simulink model "RM3_Hydraulic_PTO"  (R2019b)
settings: Solver=ode14x  StartTime=0  StopTime=100  FixedStep=0.0025  MaxStep=0.0025  RelTol=1e-3  EnableMultiTasking=on
undefined symbols (not defined in the file or in its folder): body, DiscIntNeverNeededParam, pto
libraries: fl_lib x208, sh_lib x67, nesl_utility x67, WECSim_Lib x5
(part 5 of 5)

== system RM3_Hydraulic_PTO/PTO-Sim - Crankshaft DA 4 Cylinders Try 4 WORKS /Cylinder 3/Hydraulic cylinder and valves ==
  3 Way Directional Valve : sh_lib/Valves/Directional Valves/3-Way Directional Valve  area_spec=sh.valves.directional_valves.enum.area_spec.identical  x_0_P=0 m  x_0_T=0 m  mdl_type_identical=sh.valves.directional_valves.enum.mdl_type.linear  mdl_type_different=sh.valves.directional_valves.enum.mdl_type.linear  opening_max=0.75 in  area_max=pi*(0.75/2)^2 in^2  opening_max_P_A=0.005 m  area_max_P_A=0.5e-4 m^2  opening_max_A_T=0.005 m  area_max_A_T=0.5e-4 m^2  opening_area_tab=[-.002, 0, .002, .005, .015] m  area_tab=[1e-09, 2.0352e-07, 4.0736e-05, .00011438, .00034356] m^2  opening_flow_rate_tab=[-.002, 0, .002, .005, .015] m  pressure_tab=[-10000000, -5000000, -2000000, 2000000, 5000000, 10000000] Pa  flow_rate_tab=[-1e-07, -7.0711e-08, -4.4721e-08, 4.4721e-08, 7.0711e-08, 1e-07; -2.0352e-05, -1.4391e-05, -9.1017e-06, 9.1017e-06, 1.4391e-05, 2.0352e-05; -.0040736, -.0028805, -.0018218, .0018218, .0028805, .0040736; -.011438, -.0080879, -.0051152, .0051152, .0080879, .011438; -.034356, -.024293, -.015364, .015364, .024293, .034356] m^3/s  opening_area_tab_P_A=[-.002, 0, .002, .005, .015] m  area_tab_P_A=[1e-09, 2.0352e-07, 4.0736e-05, .00011438, .00034356] m^2  opening_flow_rate_tab_P_A=[-.002, 0, .002, .005, .015] m  pressure_tab_P_A=[-10000000, -5000000, -2000000, 2000000, 5000000, 10000000] Pa  flow_rate_tab_P_A=[-1e-07, -7.0711e-08, -4.4721e-08, 4.4721e-08, 7.0711e-08, 1e-07; -2.0352e-05, -1.4391e-05, -9.1017e-06, 9.1017e-06, 1.4391e-05, 2.0352e-05; -.0040736, -.0028805, -.0018218, .0018218, .0028805, .0040736; -.011438, -.0080879, -.0051152, .0051152, .0080879, .011438; -.034356, -.024293, -.015364, .015364, .024293, .034356] m^3/s  opening_area_tab_A_T=[-.002, 0, .002, .005, .015] m  area_tab_A_T=[1e-09, 2.0352e-07, 4.0736e-05, .00011438, .00034356] m^2  opening_flow_rate_tab_A_T=[-.002, 0, .002, .005, .015] m  pressure_tab_A_T=[-10000000, -5000000, -2000000, 2000000, 5000000, 10000000] Pa  flow_rate_tab_A_T=[-1e-07, -7.0711e-08, -4.4721e-08, 4.4721e-08, 7.0711e-08, 1e-07; -2.0352e-05, -1.4391e-05, -9.1017e-06, 9.1017e-06, 1.4391e-05, 2.0352e-05; -.0040736, -.0028805, -.0018218, .0018218, .0028805, .0040736; -.011438, -.0080879, -.0051152, .0051152, .0080879, .011438; -.034356, -.024293, -.015364, .015364, .024293, .034356] m^3/s  interp_method_identical=sh.valves.directional_valves.enum.interp_method.linear  interp_method_different=sh.valves.directional_valves.enum.interp_method.linear  extrap_method_identical=sh.valves.directional_valves.enum.extrap_method.linear  extrap_method_different=sh.valves.directional_valves.enum.extrap_method.linear  A_leak=1e-12 m^2  C_d=0.7  lam_spec=sh.valves.directional_valves.enum.lam_spec.pressure_ratio  B_lam=0.999  Re_cr=12
      settings: SourceProductName=Simscape Fluids  SourceProductBaseCode=SH  InternalSimscapePortConfiguration="{\"Bottom\":[],\"Left\":[{\"id\":\"A\",\"label\":\"A\",\"type\":\"foundation.hydraulic.hydraulic\"}],\"Right\":[{\"id\":\"S\",\"label\":\"S\",\"type\":\"input\"},{\"id\":\"P\",\"label\":\"P\",\"type\":\"foundation.hydraulic.hydraulic\"},{\"id\":\"T\",\"label\":\"T\",\"type\":\"foundation.hydraulic.hydraulic\"}],\"Top\":[]}"
  3 Way Directional Valve1 : sh_lib/Valves/Directional Valves/3-Way Directional Valve  area_spec=sh.valves.directional_valves.enum.area_spec.identical  x_0_P=0 m  x_0_T=0 m  mdl_type_identical=sh.valves.directional_valves.enum.mdl_type.linear  mdl_type_different=sh.valves.directional_valves.enum.mdl_type.linear  opening_max=0.75 in  area_max=pi*(0.75/2)^2 in^2  opening_max_P_A=0.005 m  area_max_P_A=0.5e-4 m^2  opening_max_A_T=0.005 m  area_max_A_T=0.5e-4 m^2  opening_area_tab=[-.002, 0, .002, .005, .015] m  area_tab=[1e-09, 2.0352e-07, 4.0736e-05, .00011438, .00034356] m^2  opening_flow_rate_tab=[-.002, 0, .002, .005, .015] m  pressure_tab=[-10000000, -5000000, -2000000, 2000000, 5000000, 10000000] Pa  flow_rate_tab=[-1e-07, -7.0711e-08, -4.4721e-08, 4.4721e-08, 7.0711e-08, 1e-07; -2.0352e-05, -1.4391e-05, -9.1017e-06, 9.1017e-06, 1.4391e-05, 2.0352e-05; -.0040736, -.0028805, -.0018218, .0018218, .0028805, .0040736; -.011438, -.0080879, -.0051152, .0051152, .0080879, .011438; -.034356, -.024293, -.015364, .015364, .024293, .034356] m^3/s  opening_area_tab_P_A=[-.002, 0, .002, .005, .015] m  area_tab_P_A=[1e-09, 2.0352e-07, 4.0736e-05, .00011438, .00034356] m^2  opening_flow_rate_tab_P_A=[-.002, 0, .002, .005, .015] m  pressure_tab_P_A=[-10000000, -5000000, -2000000, 2000000, 5000000, 10000000] Pa  flow_rate_tab_P_A=[-1e-07, -7.0711e-08, -4.4721e-08, 4.4721e-08, 7.0711e-08, 1e-07; -2.0352e-05, -1.4391e-05, -9.1017e-06, 9.1017e-06, 1.4391e-05, 2.0352e-05; -.0040736, -.0028805, -.0018218, .0018218, .0028805, .0040736; -.011438, -.0080879, -.0051152, .0051152, .0080879, .011438; -.034356, -.024293, -.015364, .015364, .024293, .034356] m^3/s  opening_area_tab_A_T=[-.002, 0, .002, .005, .015] m  area_tab_A_T=[1e-09, 2.0352e-07, 4.0736e-05, .00011438, .00034356] m^2  opening_flow_rate_tab_A_T=[-.002, 0, .002, .005, .015] m  pressure_tab_A_T=[-10000000, -5000000, -2000000, 2000000, 5000000, 10000000] Pa  flow_rate_tab_A_T=[-1e-07, -7.0711e-08, -4.4721e-08, 4.4721e-08, 7.0711e-08, 1e-07; -2.0352e-05, -1.4391e-05, -9.1017e-06, 9.1017e-06, 1.4391e-05, 2.0352e-05; -.0040736, -.0028805, -.0018218, .0018218, .0028805, .0040736; -.011438, -.0080879, -.0051152, .0051152, .0080879, .011438; -.034356, -.024293, -.015364, .015364, .024293, .034356] m^3/s  interp_method_identical=sh.valves.directional_valves.enum.interp_method.linear  interp_method_different=sh.valves.directional_valves.enum.interp_method.linear  extrap_method_identical=sh.valves.directional_valves.enum.extrap_method.linear  extrap_method_different=sh.valves.directional_valves.enum.extrap_method.linear  A_leak=1e-12 m^2  C_d=0.7  lam_spec=sh.valves.directional_valves.enum.lam_spec.pressure_ratio  B_lam=0.999  Re_cr=12
      settings: SourceProductName=Simscape Fluids  SourceProductBaseCode=SH  InternalSimscapePortConfiguration="{\"Bottom\":[],\"Left\":[{\"id\":\"A\",\"label\":\"A\",\"type\":\"foundation.hydraulic.hydraulic\"}],\"Right\":[{\"id\":\"S\",\"label\":\"S\",\"type\":\"input\"},{\"id\":\"P\",\"label\":\"P\",\"type\":\"foundation.hydraulic.hydraulic\"},{\"id\":\"T\",\"label\":\"T\",\"type\":\"foundation.hydraulic.hydraulic\"}],\"Top\":[]}"
  Check Valve : sh_lib/Valves/Directional Valves/Check Valve  Commented=on  area_max=pi*(0.75/2)^2 in^2  pres_crack=0.3e5 Pa  pres_max=1.2e5 Pa  C_d=0.7  A_leak=1e-12 m^2  lam_spec=1  B_lam=0.999  Re_cr=12  dynamic=0  tau=0.1 s  area_init=1e-12 m^2
      settings: SourceProductName=Simscape Fluids  SourceProductBaseCode=SH  InternalSimscapePortConfiguration="{\"Bottom\":[],\"Left\":[{\"id\":\"A\",\"label\":\"A\",\"type\":\"foundation.hydraulic.hydraulic\"}],\"Right\":[{\"id\":\"B\",\"label\":\"B\",\"type\":\"foundation.hydraulic.hydraulic\"}],\"Top\":[]}"
  Check Valve1 : sh_lib/Valves/Directional Valves/Check Valve  Commented=on  area_max=pi*(0.75/2)^2 in^2  pres_crack=0.3e5 Pa  pres_max=1.2e5 Pa  C_d=0.7  A_leak=1e-12 m^2  lam_spec=1  B_lam=0.999  Re_cr=12  dynamic=0  tau=0.1 s  area_init=1e-12 m^2
      settings: SourceProductName=Simscape Fluids  SourceProductBaseCode=SH  InternalSimscapePortConfiguration="{\"Bottom\":[],\"Left\":[{\"id\":\"A\",\"label\":\"A\",\"type\":\"foundation.hydraulic.hydraulic\"}],\"Right\":[{\"id\":\"B\",\"label\":\"B\",\"type\":\"foundation.hydraulic.hydraulic\"}],\"Top\":[]}"
  Double-Acting Hydraulic Cylinder (Simple) : sh_lib/Hydraulic Cylinders/Double-Acting Hydraulic Cylinder (Simple)  area_A=0.0025746658/4 m^2  area_B=0.0025746658/4 m^2  stroke=12 in  init_pos=5 in  penetr_coeff=1e12 s*N/m^2  or=1
      settings: SourceProductName=Simscape Fluids  SourceProductBaseCode=SH  InternalSimscapePortConfiguration="{\"Bottom\":[],\"Left\":[{\"id\":\"C\",\"label\":\"C\",\"type\":\"foundation.mechanical.translational.translational\"},{\"id\":\"A\",\"label\":\"A\",\"type\":\"foundation.hydraulic.hydraulic\"}],\"Right\":[{\"id\":\"R\",\"label\":\"R\",\"type\":\"foundation.mechanical.translational.translational\"},{\"id\":\"B\",\"label\":\"B\",\"type\":\"foundation.hydraulic.hydraulic\"}],\"Top\":[]}"
  Ideal Force Sensor : fl_lib/Mechanical/Mechanical Sensors/Ideal Force Sensor
  Ideal Translational Velocity Source : fl_lib/Mechanical/Mechanical Sources/Ideal Translational Velocity Source
  Mechanical Translational Reference : fl_lib/Mechanical/Translational Elements/Mechanical Translational Reference
  Mechanical Translational Reference1 : fl_lib/Mechanical/Translational Elements/Mechanical Translational Reference
  PS Gain : fl_lib/Physical Signals/Functions/PS Gain  gain=-1
  PS-Simulink Converter : nesl_utility/PS-Simulink Converter  PhysicalDomain=network_engine_domain  SubClassName=ps_output  LeftPortType=input  RightPortType=output  PseudoPeriodic=off  Frequencies=[]  Unit=N  AffineConversion=off
  PS-Simulink Converter2 : nesl_utility/PS-Simulink Converter  PhysicalDomain=network_engine_domain  SubClassName=ps_output  LeftPortType=input  RightPortType=output  PseudoPeriodic=off  Frequencies=[]  Unit=inherit  AffineConversion=off
  Relay : Relay  OnSwitchValue=0  OffSwitchValue=0  OffOutputValue=-1
  Simulink-PS Converter1 : nesl_utility/Simulink-PS Converter  PhysicalDomain=network_engine_domain  SubClassName=ps_input  LeftPortType=input  RightPortType=output  PseudoPeriodic=off  Frequencies=[]  NoiseDistribution=none  NoiseParameters=[]  Unit=1  AffineConversion=off  FilteringAndDerivatives=zero  SimscapeFilterOrder=1  InputFilterTimeConstant=0.001  UdotUserProvided=0
  Velocity input : PMIOPort  Side=Left
  Flow out : PMIOPort  Port=2  Side=Left
  Seawater In : PMIOPort  Port=3  Side=Left
  Force Out : Outport
  wires:
  PS-Simulink Converter2/1 -> Relay/1
  Relay/1 -> Simulink-PS Converter1/1
  PS-Simulink Converter/1 -> Force Out/1
  connections:
  Ideal Translational Velocity Source/LConn1 -- Double-Acting Hydraulic Cylinder (Simple)/RConn1
  3 Way Directional Valve1/RConn2 -- 3 Way Directional Valve/RConn2 -- Seawater In/RConn1
  3 Way Directional Valve/RConn3 -- 3 Way Directional Valve1/RConn3 -- Flow out/RConn1
  3 Way Directional Valve/LConn1 -- Double-Acting Hydraulic Cylinder (Simple)/LConn2
  Simulink-PS Converter1/RConn1 -- PS Gain/LConn1 -- 3 Way Directional Valve/RConn1
  Ideal Translational Velocity Source/RConn1 -- PS-Simulink Converter2/LConn1 -- Velocity input/RConn1
  Ideal Translational Velocity Source/RConn2 -- Mechanical Translational Reference1/LConn1
  Double-Acting Hydraulic Cylinder (Simple)/RConn2 -- 3 Way Directional Valve1/LConn1
  PS Gain/RConn1 -- 3 Way Directional Valve1/RConn1
  Ideal Force Sensor/RConn2 -- PS-Simulink Converter/LConn1
  Ideal Force Sensor/RConn1 -- Mechanical Translational Reference/LConn1
  Ideal Force Sensor/LConn1 -- Double-Acting Hydraulic Cylinder (Simple)/LConn1

== system RM3_Hydraulic_PTO/PTO-Sim - Crankshaft DA 4 Cylinders Try 4 WORKS /Cylinder 4/Cylinder 1 to PTO Force convert ==
  Crank radius : Inport
  Crank initial angle : Inport  Port=2
  Angle disp : Inport  Port=3
  Spool radius : Inport  Port=4
  Cylinder Force : Inport  Port=5
  Constant : Constant
  Divide1 : Product  Inputs=*/
  Mod angle : Constant  Value=2*pi
  PTO Force Cylinder 1 : Product  Inputs=4
  Sin(theta) : Trigonometry
  Sum : Sum  Inputs=|++
  To get Theta : Math  Operator=mod  SignedPower=off  SaturateOnIntegerOverflow=on
  Theta : Outport
  sing(theta) : Outport  Port=2
  PTO Force Cyl : Outport  Port=3
  wires:
  Mod angle/1 -> To get Theta/2
  Angle disp/1 -> Sum/2
  To get Theta/1 -> Theta/1, Sin(theta)/1
  PTO Force Cylinder 1/1 -> PTO Force Cyl/1
  Divide1/1 -> PTO Force Cylinder 1/3
  Sin(theta)/1 -> sing(theta)/1, PTO Force Cylinder 1/2
  Constant/1 -> Divide1/1
  Crank initial angle/1 -> Sum/1
  Sum/1 -> To get Theta/1
  Spool radius/1 -> Divide1/2
  Cylinder Force/1 -> PTO Force Cylinder 1/4
  Crank radius/1 -> PTO Force Cylinder 1/1

== system RM3_Hydraulic_PTO/PTO-Sim - Crankshaft DA 4 Cylinders Try 4 WORKS /Cylinder 4/Hydraulic cylinder and valves ==
  3 Way Directional Valve : sh_lib/Valves/Directional Valves/3-Way Directional Valve  area_spec=sh.valves.directional_valves.enum.area_spec.identical  x_0_P=0 m  x_0_T=0 m  mdl_type_identical=sh.valves.directional_valves.enum.mdl_type.linear  mdl_type_different=sh.valves.directional_valves.enum.mdl_type.linear  opening_max=0.75 in  area_max=pi*(0.75/2)^2 in^2  opening_max_P_A=0.005 m  area_max_P_A=0.5e-4 m^2  opening_max_A_T=0.005 m  area_max_A_T=0.5e-4 m^2  opening_area_tab=[-.002, 0, .002, .005, .015] m  area_tab=[1e-09, 2.0352e-07, 4.0736e-05, .00011438, .00034356] m^2  opening_flow_rate_tab=[-.002, 0, .002, .005, .015] m  pressure_tab=[-10000000, -5000000, -2000000, 2000000, 5000000, 10000000] Pa  flow_rate_tab=[-1e-07, -7.0711e-08, -4.4721e-08, 4.4721e-08, 7.0711e-08, 1e-07; -2.0352e-05, -1.4391e-05, -9.1017e-06, 9.1017e-06, 1.4391e-05, 2.0352e-05; -.0040736, -.0028805, -.0018218, .0018218, .0028805, .0040736; -.011438, -.0080879, -.0051152, .0051152, .0080879, .011438; -.034356, -.024293, -.015364, .015364, .024293, .034356] m^3/s  opening_area_tab_P_A=[-.002, 0, .002, .005, .015] m  area_tab_P_A=[1e-09, 2.0352e-07, 4.0736e-05, .00011438, .00034356] m^2  opening_flow_rate_tab_P_A=[-.002, 0, .002, .005, .015] m  pressure_tab_P_A=[-10000000, -5000000, -2000000, 2000000, 5000000, 10000000] Pa  flow_rate_tab_P_A=[-1e-07, -7.0711e-08, -4.4721e-08, 4.4721e-08, 7.0711e-08, 1e-07; -2.0352e-05, -1.4391e-05, -9.1017e-06, 9.1017e-06, 1.4391e-05, 2.0352e-05; -.0040736, -.0028805, -.0018218, .0018218, .0028805, .0040736; -.011438, -.0080879, -.0051152, .0051152, .0080879, .011438; -.034356, -.024293, -.015364, .015364, .024293, .034356] m^3/s  opening_area_tab_A_T=[-.002, 0, .002, .005, .015] m  area_tab_A_T=[1e-09, 2.0352e-07, 4.0736e-05, .00011438, .00034356] m^2  opening_flow_rate_tab_A_T=[-.002, 0, .002, .005, .015] m  pressure_tab_A_T=[-10000000, -5000000, -2000000, 2000000, 5000000, 10000000] Pa  flow_rate_tab_A_T=[-1e-07, -7.0711e-08, -4.4721e-08, 4.4721e-08, 7.0711e-08, 1e-07; -2.0352e-05, -1.4391e-05, -9.1017e-06, 9.1017e-06, 1.4391e-05, 2.0352e-05; -.0040736, -.0028805, -.0018218, .0018218, .0028805, .0040736; -.011438, -.0080879, -.0051152, .0051152, .0080879, .011438; -.034356, -.024293, -.015364, .015364, .024293, .034356] m^3/s  interp_method_identical=sh.valves.directional_valves.enum.interp_method.linear  interp_method_different=sh.valves.directional_valves.enum.interp_method.linear  extrap_method_identical=sh.valves.directional_valves.enum.extrap_method.linear  extrap_method_different=sh.valves.directional_valves.enum.extrap_method.linear  A_leak=1e-12 m^2  C_d=0.7  lam_spec=sh.valves.directional_valves.enum.lam_spec.pressure_ratio  B_lam=0.999  Re_cr=12
      settings: SourceProductName=Simscape Fluids  SourceProductBaseCode=SH  InternalSimscapePortConfiguration="{\"Bottom\":[],\"Left\":[{\"id\":\"A\",\"label\":\"A\",\"type\":\"foundation.hydraulic.hydraulic\"}],\"Right\":[{\"id\":\"S\",\"label\":\"S\",\"type\":\"input\"},{\"id\":\"P\",\"label\":\"P\",\"type\":\"foundation.hydraulic.hydraulic\"},{\"id\":\"T\",\"label\":\"T\",\"type\":\"foundation.hydraulic.hydraulic\"}],\"Top\":[]}"
  3 Way Directional Valve1 : sh_lib/Valves/Directional Valves/3-Way Directional Valve  area_spec=sh.valves.directional_valves.enum.area_spec.identical  x_0_P=0 m  x_0_T=0 m  mdl_type_identical=sh.valves.directional_valves.enum.mdl_type.linear  mdl_type_different=sh.valves.directional_valves.enum.mdl_type.linear  opening_max=0.75 in  area_max=pi*(0.75/2)^2 in^2  opening_max_P_A=0.005 m  area_max_P_A=0.5e-4 m^2  opening_max_A_T=0.005 m  area_max_A_T=0.5e-4 m^2  opening_area_tab=[-.002, 0, .002, .005, .015] m  area_tab=[1e-09, 2.0352e-07, 4.0736e-05, .00011438, .00034356] m^2  opening_flow_rate_tab=[-.002, 0, .002, .005, .015] m  pressure_tab=[-10000000, -5000000, -2000000, 2000000, 5000000, 10000000] Pa  flow_rate_tab=[-1e-07, -7.0711e-08, -4.4721e-08, 4.4721e-08, 7.0711e-08, 1e-07; -2.0352e-05, -1.4391e-05, -9.1017e-06, 9.1017e-06, 1.4391e-05, 2.0352e-05; -.0040736, -.0028805, -.0018218, .0018218, .0028805, .0040736; -.011438, -.0080879, -.0051152, .0051152, .0080879, .011438; -.034356, -.024293, -.015364, .015364, .024293, .034356] m^3/s  opening_area_tab_P_A=[-.002, 0, .002, .005, .015] m  area_tab_P_A=[1e-09, 2.0352e-07, 4.0736e-05, .00011438, .00034356] m^2  opening_flow_rate_tab_P_A=[-.002, 0, .002, .005, .015] m  pressure_tab_P_A=[-10000000, -5000000, -2000000, 2000000, 5000000, 10000000] Pa  flow_rate_tab_P_A=[-1e-07, -7.0711e-08, -4.4721e-08, 4.4721e-08, 7.0711e-08, 1e-07; -2.0352e-05, -1.4391e-05, -9.1017e-06, 9.1017e-06, 1.4391e-05, 2.0352e-05; -.0040736, -.0028805, -.0018218, .0018218, .0028805, .0040736; -.011438, -.0080879, -.0051152, .0051152, .0080879, .011438; -.034356, -.024293, -.015364, .015364, .024293, .034356] m^3/s  opening_area_tab_A_T=[-.002, 0, .002, .005, .015] m  area_tab_A_T=[1e-09, 2.0352e-07, 4.0736e-05, .00011438, .00034356] m^2  opening_flow_rate_tab_A_T=[-.002, 0, .002, .005, .015] m  pressure_tab_A_T=[-10000000, -5000000, -2000000, 2000000, 5000000, 10000000] Pa  flow_rate_tab_A_T=[-1e-07, -7.0711e-08, -4.4721e-08, 4.4721e-08, 7.0711e-08, 1e-07; -2.0352e-05, -1.4391e-05, -9.1017e-06, 9.1017e-06, 1.4391e-05, 2.0352e-05; -.0040736, -.0028805, -.0018218, .0018218, .0028805, .0040736; -.011438, -.0080879, -.0051152, .0051152, .0080879, .011438; -.034356, -.024293, -.015364, .015364, .024293, .034356] m^3/s  interp_method_identical=sh.valves.directional_valves.enum.interp_method.linear  interp_method_different=sh.valves.directional_valves.enum.interp_method.linear  extrap_method_identical=sh.valves.directional_valves.enum.extrap_method.linear  extrap_method_different=sh.valves.directional_valves.enum.extrap_method.linear  A_leak=1e-12 m^2  C_d=0.7  lam_spec=sh.valves.directional_valves.enum.lam_spec.pressure_ratio  B_lam=0.999  Re_cr=12
      settings: SourceProductName=Simscape Fluids  SourceProductBaseCode=SH  InternalSimscapePortConfiguration="{\"Bottom\":[],\"Left\":[{\"id\":\"A\",\"label\":\"A\",\"type\":\"foundation.hydraulic.hydraulic\"}],\"Right\":[{\"id\":\"S\",\"label\":\"S\",\"type\":\"input\"},{\"id\":\"P\",\"label\":\"P\",\"type\":\"foundation.hydraulic.hydraulic\"},{\"id\":\"T\",\"label\":\"T\",\"type\":\"foundation.hydraulic.hydraulic\"}],\"Top\":[]}"
  Check Valve : sh_lib/Valves/Directional Valves/Check Valve  Commented=on  area_max=pi*(0.75/2)^2 in^2  pres_crack=0.3e5 Pa  pres_max=1.2e5 Pa  C_d=0.7  A_leak=1e-12 m^2  lam_spec=1  B_lam=0.999  Re_cr=12  dynamic=0  tau=0.1 s  area_init=1e-12 m^2
      settings: SourceProductName=Simscape Fluids  SourceProductBaseCode=SH  InternalSimscapePortConfiguration="{\"Bottom\":[],\"Left\":[{\"id\":\"A\",\"label\":\"A\",\"type\":\"foundation.hydraulic.hydraulic\"}],\"Right\":[{\"id\":\"B\",\"label\":\"B\",\"type\":\"foundation.hydraulic.hydraulic\"}],\"Top\":[]}"
  Check Valve1 : sh_lib/Valves/Directional Valves/Check Valve  Commented=on  area_max=pi*(0.75/2)^2 in^2  pres_crack=0.3e5 Pa  pres_max=1.2e5 Pa  C_d=0.7  A_leak=1e-12 m^2  lam_spec=1  B_lam=0.999  Re_cr=12  dynamic=0  tau=0.1 s  area_init=1e-12 m^2
      settings: SourceProductName=Simscape Fluids  SourceProductBaseCode=SH  InternalSimscapePortConfiguration="{\"Bottom\":[],\"Left\":[{\"id\":\"A\",\"label\":\"A\",\"type\":\"foundation.hydraulic.hydraulic\"}],\"Right\":[{\"id\":\"B\",\"label\":\"B\",\"type\":\"foundation.hydraulic.hydraulic\"}],\"Top\":[]}"
  Double-Acting Hydraulic Cylinder (Simple) : sh_lib/Hydraulic Cylinders/Double-Acting Hydraulic Cylinder (Simple)  area_A=0.0025746658/4 m^2  area_B=0.0025746658/4 m^2  stroke=12 in  init_pos=0.5 in  penetr_coeff=1e12 s*N/m^2  or=1
      settings: SourceProductName=Simscape Fluids  SourceProductBaseCode=SH  InternalSimscapePortConfiguration="{\"Bottom\":[],\"Left\":[{\"id\":\"C\",\"label\":\"C\",\"type\":\"foundation.mechanical.translational.translational\"},{\"id\":\"A\",\"label\":\"A\",\"type\":\"foundation.hydraulic.hydraulic\"}],\"Right\":[{\"id\":\"R\",\"label\":\"R\",\"type\":\"foundation.mechanical.translational.translational\"},{\"id\":\"B\",\"label\":\"B\",\"type\":\"foundation.hydraulic.hydraulic\"}],\"Top\":[]}"
  Ideal Force Sensor : fl_lib/Mechanical/Mechanical Sensors/Ideal Force Sensor
  Ideal Translational Velocity Source : fl_lib/Mechanical/Mechanical Sources/Ideal Translational Velocity Source
  Mechanical Translational Reference : fl_lib/Mechanical/Translational Elements/Mechanical Translational Reference
  Mechanical Translational Reference1 : fl_lib/Mechanical/Translational Elements/Mechanical Translational Reference
  PS Gain : fl_lib/Physical Signals/Functions/PS Gain  gain=-1
  PS-Simulink Converter : nesl_utility/PS-Simulink Converter  PhysicalDomain=network_engine_domain  SubClassName=ps_output  LeftPortType=input  RightPortType=output  PseudoPeriodic=off  Frequencies=[]  Unit=N  AffineConversion=off
  PS-Simulink Converter2 : nesl_utility/PS-Simulink Converter  PhysicalDomain=network_engine_domain  SubClassName=ps_output  LeftPortType=input  RightPortType=output  PseudoPeriodic=off  Frequencies=[]  Unit=inherit  AffineConversion=off
  Relay : Relay  OnSwitchValue=0  OffSwitchValue=0  OffOutputValue=-1
  Simulink-PS Converter1 : nesl_utility/Simulink-PS Converter  PhysicalDomain=network_engine_domain  SubClassName=ps_input  LeftPortType=input  RightPortType=output  PseudoPeriodic=off  Frequencies=[]  NoiseDistribution=none  NoiseParameters=[]  Unit=1  AffineConversion=off  FilteringAndDerivatives=zero  SimscapeFilterOrder=1  InputFilterTimeConstant=0.001  UdotUserProvided=0
  Velocity input : PMIOPort  Side=Left
  Flow out : PMIOPort  Port=2  Side=Left
  Seawater In : PMIOPort  Port=3  Side=Left
  Force Out : Outport
  wires:
  PS-Simulink Converter2/1 -> Relay/1
  Relay/1 -> Simulink-PS Converter1/1
  PS-Simulink Converter/1 -> Force Out/1
  connections:
  Ideal Translational Velocity Source/LConn1 -- Double-Acting Hydraulic Cylinder (Simple)/RConn1
  3 Way Directional Valve1/RConn2 -- 3 Way Directional Valve/RConn2 -- Seawater In/RConn1
  3 Way Directional Valve/RConn3 -- 3 Way Directional Valve1/RConn3 -- Flow out/RConn1
  3 Way Directional Valve/LConn1 -- Double-Acting Hydraulic Cylinder (Simple)/LConn2
  Simulink-PS Converter1/RConn1 -- PS Gain/LConn1 -- 3 Way Directional Valve/RConn1
  Ideal Translational Velocity Source/RConn1 -- PS-Simulink Converter2/LConn1 -- Velocity input/RConn1
  Ideal Translational Velocity Source/RConn2 -- Mechanical Translational Reference1/LConn1
  Double-Acting Hydraulic Cylinder (Simple)/RConn2 -- 3 Way Directional Valve1/LConn1
  PS Gain/RConn1 -- 3 Way Directional Valve1/RConn1
  Ideal Force Sensor/RConn2 -- PS-Simulink Converter/LConn1
  Ideal Force Sensor/RConn1 -- Mechanical Translational Reference/LConn1
  Ideal Force Sensor/LConn1 -- Double-Acting Hydraulic Cylinder (Simple)/LConn1
